simulink model "PassengerCar"  (R2019b)
settings: Solver=ode1  StartTime=0  StopTime=25  FixedStep=1.0000000000000000e-003  RelTol=1e-3
InitFcn:
  | sampleTime = str2double(get_param(bdroot, 'FixedStep'));
undefined symbols (not defined in the file or in its folder): AccPedalPos, BrakePedalPos, BrakeSwitch, DiscIntNeverNeededParam, DYNA4, EngSpd, IgnitionSwitch, InitialGear, InitialSpeed, IntendedEngTrq, LeftIndicator, MainBrakePress, MaxGear, MDL, MinGear, RefAcc, RefLane, RefLatPos, RefPath, RefPathCurv, RefSpd, RefSpdPreview, RefSpdRetrospect, RightIndicator, SteeringWheelAng, SteeringWheelTrq, UserDefinedRefValue, vm_const
libraries: UtilitiesLibrary x31, simulink x18, WheelSystemModules x13, LongitudinalControllerModules x13, LateralControllerModules x7, AnimationBusselectorModules x5, EnvironmentModules x5, BasicEngineControlModules x5, MiscellaneousControlModules x5, Animation3Modules x4, AuxiliariesModules x4, TireModules x4
(part 38 of 39)

== system PassengerCar/Vehicle/Drivetrain/DrivetrainPhysics/DrivetrainPhysicsOutputs/Rear3RightShaftOutput/Rear3RightShaftOutput ==
  Trq[Nm]___UNIQUE_1 : Inport  Description=|  PortDimensions=[1]
      | <name>Trq[Nm]</name>
      | <comment></comment>
  RotSpdDifferentialOut[rad/s]___UNIQUE_1 : Inport  Description=|  Port=2  PortDimensions=[1]
      | <name>RotSpdDifferentialOut[rad/s]</name>
      | <comment></comment>
  RotAcc[rad/s**2]___UNIQUE_1 : Inport  Description=|  Port=3  PortDimensions=[1]
      | <name>RotAcc[rad/s**2]</name>
      | <comment></comment>
  DerivativeOfTrq_wrt_RotAng[Nm/rad]___UNIQUE_1 : Inport  Description=|  Port=4  PortDimensions=[1]
      | <name>DerivativeOfTrq_wrt_RotAng[Nm/rad]</name>
      | <comment></comment>
  DerivativeOfTrq_wrt_WheelSpd[Nm/(rad/s)]___UNIQUE_1 : Inport  Description=|  Port=5  PortDimensions=[1]
      | <name>DerivativeOfTrq_wrt_WheelSpd[Nm/(rad/s)]</name>
      | <comment></comment>
  AddInrt[kg*m**2]___UNIQUE_1 : Inport  Description=|  Port=6  PortDimensions=[1]
      | <name>AddInrt[kg*m**2]</name>
      | <comment></comment>
  FrictionTrq[Nm]___UNIQUE_1 : Inport  Description=|  Port=7  PortDimensions=[1]
      | <name>FrictionTrq[Nm]</name>
      | <comment></comment>
  __TDD__Rear3RightShaft.AddInrt[kg*m**2] : Demux  Outputs=[1]
  __TDD__Rear3RightShaft.DerivativeOfTrq_wrt_RotAng[Nm/rad] : Demux  Outputs=[1]
  __TDD__Rear3RightShaft.DerivativeOfTrq_wrt_WheelSpd[Nm/(rad/s)] : Demux  Outputs=[1]
  __TDD__Rear3RightShaft.FrictionTrq[Nm] : Demux  Outputs=[1]
  __TDD__Rear3RightShaft.RotAcc[rad/s**2] : Demux  Outputs=[1]
  __TDD__Rear3RightShaft.RotSpdDifferentialOut[rad/s] : Demux  Outputs=[1]
  __TDD__Rear3RightShaft.Trq[Nm] : Demux  Outputs=[1]
  __TDO__Rear3RightShaft : BusCreator  Inputs=7
  Rear3RightShaft___UNIQUE_1 : Outport  Description=|  PortDimensions=[7]  VectorParamsAs1DForOutWhenUnconnected=off
      | <name>Trq[Nm]</name>
      | <comment></comment>
  wires:
  Trq[Nm]___UNIQUE_1/1 -> __TDD__Rear3RightShaft.Trq[Nm]/1
  __TDD__Rear3RightShaft.Trq[Nm]/1 -> __TDO__Rear3RightShaft/1  "Trq[Nm]"
  RotSpdDifferentialOut[rad/s]___UNIQUE_1/1 -> __TDD__Rear3RightShaft.RotSpdDifferentialOut[rad/s]/1
  __TDD__Rear3RightShaft.RotSpdDifferentialOut[rad/s]/1 -> __TDO__Rear3RightShaft/2  "RotSpdDifferentialOut[rad/s]"
  RotAcc[rad/s**2]___UNIQUE_1/1 -> __TDD__Rear3RightShaft.RotAcc[rad/s**2]/1
  __TDD__Rear3RightShaft.RotAcc[rad/s**2]/1 -> __TDO__Rear3RightShaft/3  "RotAcc[rad/s**2]"
  DerivativeOfTrq_wrt_RotAng[Nm/rad]___UNIQUE_1/1 -> __TDD__Rear3RightShaft.DerivativeOfTrq_wrt_RotAng[Nm/rad]/1
  __TDD__Rear3RightShaft.DerivativeOfTrq_wrt_RotAng[Nm/rad]/1 -> __TDO__Rear3RightShaft/4  "DerivativeOfTrq_wrt_RotAng[Nm/rad]"
  DerivativeOfTrq_wrt_WheelSpd[Nm/(rad/s)]___UNIQUE_1/1 -> __TDD__Rear3RightShaft.DerivativeOfTrq_wrt_WheelSpd[Nm/(rad/s)]/1
  __TDD__Rear3RightShaft.DerivativeOfTrq_wrt_WheelSpd[Nm/(rad/s)]/1 -> __TDO__Rear3RightShaft/5  "DerivativeOfTrq_wrt_WheelSpd[Nm/(rad/s)]"
  AddInrt[kg*m**2]___UNIQUE_1/1 -> __TDD__Rear3RightShaft.AddInrt[kg*m**2]/1
  __TDD__Rear3RightShaft.AddInrt[kg*m**2]/1 -> __TDO__Rear3RightShaft/6  "AddInrt[kg*m**2]"
  FrictionTrq[Nm]___UNIQUE_1/1 -> __TDD__Rear3RightShaft.FrictionTrq[Nm]/1
  __TDD__Rear3RightShaft.FrictionTrq[Nm]/1 -> __TDO__Rear3RightShaft/7  "FrictionTrq[Nm]"
  __TDO__Rear3RightShaft/1 -> Rear3RightShaft___UNIQUE_1/1  "Rear3RightShaft"

== system PassengerCar/Vehicle/Drivetrain/DrivetrainPhysics/DrivetrainPhysicsOutputs/RearDifferentialOutput/RearDifferentialOutput ==
  InSpd[rad/s]___UNIQUE_1 : Inport  Description=|  PortDimensions=[1]
      | <name>InSpd[rad/s]</name>
      | <comment></comment>
  LeftOutCutTrq[Nm]___UNIQUE_1 : Inport  Description=|  Port=2  PortDimensions=[1]
      | <name>LeftOutCutTrq[Nm]</name>
      | <comment></comment>
  RightOutCutTrq[Nm]___UNIQUE_1 : Inport  Description=|  Port=3  PortDimensions=[1]
      | <name>RightOutCutTrq[Nm]</name>
      | <comment></comment>
  LossPower[W]___UNIQUE_1 : Inport  Description=|  Port=4  PortDimensions=[1]
      | <name>LossPower[W]</name>
      | <comment></comment>
  __TDD__RearDifferential.InSpd[rad/s] : Demux  Outputs=[1]
  __TDD__RearDifferential.LeftOutCutTrq[Nm] : Demux  Outputs=[1]
  __TDD__RearDifferential.LossPower[W] : Demux  Outputs=[1]
  __TDD__RearDifferential.RightOutCutTrq[Nm] : Demux  Outputs=[1]
  __TDO__RearDifferential : BusCreator  Inputs=4
  RearDifferential___UNIQUE_1 : Outport  Description=|  PortDimensions=[4]  VectorParamsAs1DForOutWhenUnconnected=off
      | <name>InSpd[rad/s]</name>
      | <comment></comment>
  wires:
  InSpd[rad/s]___UNIQUE_1/1 -> __TDD__RearDifferential.InSpd[rad/s]/1
  __TDD__RearDifferential.InSpd[rad/s]/1 -> __TDO__RearDifferential/1  "InSpd[rad/s]"
  LeftOutCutTrq[Nm]___UNIQUE_1/1 -> __TDD__RearDifferential.LeftOutCutTrq[Nm]/1
  __TDD__RearDifferential.LeftOutCutTrq[Nm]/1 -> __TDO__RearDifferential/2  "LeftOutCutTrq[Nm]"
  RightOutCutTrq[Nm]___UNIQUE_1/1 -> __TDD__RearDifferential.RightOutCutTrq[Nm]/1
  __TDD__RearDifferential.RightOutCutTrq[Nm]/1 -> __TDO__RearDifferential/3  "RightOutCutTrq[Nm]"
  LossPower[W]___UNIQUE_1/1 -> __TDD__RearDifferential.LossPower[W]/1
  __TDD__RearDifferential.LossPower[W]/1 -> __TDO__RearDifferential/4  "LossPower[W]"
  __TDO__RearDifferential/1 -> RearDifferential___UNIQUE_1/1  "RearDifferential"

== system PassengerCar/Vehicle/Drivetrain/DrivetrainPhysics/DrivetrainPhysicsOutputs/RearLeftShaftOutput/RearLeftShaftOutput ==
  Trq[Nm]___UNIQUE_1 : Inport  Description=|  PortDimensions=[1]
      | <name>Trq[Nm]</name>
      | <comment></comment>
  RotSpdDifferentialOut[rad/s]___UNIQUE_1 : Inport  Description=|  Port=2  PortDimensions=[1]
      | <name>RotSpdDifferentialOut[rad/s]</name>
      | <comment></comment>
  RotAcc[rad/s**2]___UNIQUE_1 : Inport  Description=|  Port=3  PortDimensions=[1]
      | <name>RotAcc[rad/s**2]</name>
      | <comment></comment>
  DerivativeOfTrq_wrt_RotAng[Nm/rad]___UNIQUE_1 : Inport  Description=|  Port=4  PortDimensions=[1]
      | <name>DerivativeOfTrq_wrt_RotAng[Nm/rad]</name>
      | <comment></comment>
  DerivativeOfTrq_wrt_WheelSpd[Nm/(rad/s)]___UNIQUE_1 : Inport  Description=|  Port=5  PortDimensions=[1]
      | <name>DerivativeOfTrq_wrt_WheelSpd[Nm/(rad/s)]</name>
      | <comment></comment>
  AddInrt[kg*m**2]___UNIQUE_1 : Inport  Description=|  Port=6  PortDimensions=[1]
      | <name>AddInrt[kg*m**2]</name>
      | <comment></comment>
  FrictionTrq[Nm]___UNIQUE_1 : Inport  Description=|  Port=7  PortDimensions=[1]
      | <name>FrictionTrq[Nm]</name>
      | <comment></comment>
  __TDD__RearLeftShaft.AddInrt[kg*m**2] : Demux  Outputs=[1]
  __TDD__RearLeftShaft.DerivativeOfTrq_wrt_RotAng[Nm/rad] : Demux  Outputs=[1]
  __TDD__RearLeftShaft.DerivativeOfTrq_wrt_WheelSpd[Nm/(rad/s)] : Demux  Outputs=[1]
  __TDD__RearLeftShaft.FrictionTrq[Nm] : Demux  Outputs=[1]
  __TDD__RearLeftShaft.RotAcc[rad/s**2] : Demux  Outputs=[1]
  __TDD__RearLeftShaft.RotSpdDifferentialOut[rad/s] : Demux  Outputs=[1]
  __TDD__RearLeftShaft.Trq[Nm] : Demux  Outputs=[1]
  __TDO__RearLeftShaft : BusCreator  Inputs=7
  RearLeftShaft___UNIQUE_1 : Outport  Description=|  PortDimensions=[7]  VectorParamsAs1DForOutWhenUnconnected=off
      | <name>Trq[Nm]</name>
      | <comment></comment>
  wires:
  Trq[Nm]___UNIQUE_1/1 -> __TDD__RearLeftShaft.Trq[Nm]/1
  __TDD__RearLeftShaft.Trq[Nm]/1 -> __TDO__RearLeftShaft/1  "Trq[Nm]"
  RotSpdDifferentialOut[rad/s]___UNIQUE_1/1 -> __TDD__RearLeftShaft.RotSpdDifferentialOut[rad/s]/1
  __TDD__RearLeftShaft.RotSpdDifferentialOut[rad/s]/1 -> __TDO__RearLeftShaft/2  "RotSpdDifferentialOut[rad/s]"
  RotAcc[rad/s**2]___UNIQUE_1/1 -> __TDD__RearLeftShaft.RotAcc[rad/s**2]/1
  __TDD__RearLeftShaft.RotAcc[rad/s**2]/1 -> __TDO__RearLeftShaft/3  "RotAcc[rad/s**2]"
  DerivativeOfTrq_wrt_RotAng[Nm/rad]___UNIQUE_1/1 -> __TDD__RearLeftShaft.DerivativeOfTrq_wrt_RotAng[Nm/rad]/1
  __TDD__RearLeftShaft.DerivativeOfTrq_wrt_RotAng[Nm/rad]/1 -> __TDO__RearLeftShaft/4  "DerivativeOfTrq_wrt_RotAng[Nm/rad]"
  DerivativeOfTrq_wrt_WheelSpd[Nm/(rad/s)]___UNIQUE_1/1 -> __TDD__RearLeftShaft.DerivativeOfTrq_wrt_WheelSpd[Nm/(rad/s)]/1
  __TDD__RearLeftShaft.DerivativeOfTrq_wrt_WheelSpd[Nm/(rad/s)]/1 -> __TDO__RearLeftShaft/5  "DerivativeOfTrq_wrt_WheelSpd[Nm/(rad/s)]"
  AddInrt[kg*m**2]___UNIQUE_1/1 -> __TDD__RearLeftShaft.AddInrt[kg*m**2]/1
  __TDD__RearLeftShaft.AddInrt[kg*m**2]/1 -> __TDO__RearLeftShaft/6  "AddInrt[kg*m**2]"
  FrictionTrq[Nm]___UNIQUE_1/1 -> __TDD__RearLeftShaft.FrictionTrq[Nm]/1
  __TDD__RearLeftShaft.FrictionTrq[Nm]/1 -> __TDO__RearLeftShaft/7  "FrictionTrq[Nm]"
  __TDO__RearLeftShaft/1 -> RearLeftShaft___UNIQUE_1/1  "RearLeftShaft"

== system PassengerCar/Vehicle/Drivetrain/DrivetrainPhysics/DrivetrainPhysicsOutputs/RearRightShaftOutput/RearRightShaftOutput ==
  Trq[Nm]___UNIQUE_1 : Inport  Description=|  PortDimensions=[1]
      | <name>Trq[Nm]</name>
      | <comment></comment>
  RotSpdDifferentialOut[rad/s]___UNIQUE_1 : Inport  Description=|  Port=2  PortDimensions=[1]
      | <name>RotSpdDifferentialOut[rad/s]</name>
      | <comment></comment>
  RotAcc[rad/s**2]___UNIQUE_1 : Inport  Description=|  Port=3  PortDimensions=[1]
      | <name>RotAcc[rad/s**2]</name>
      | <comment></comment>
  DerivativeOfTrq_wrt_RotAng[Nm/rad]___UNIQUE_1 : Inport  Description=|  Port=4  PortDimensions=[1]
      | <name>DerivativeOfTrq_wrt_RotAng[Nm/rad]</name>
      | <comment></comment>
  DerivativeOfTrq_wrt_WheelSpd[Nm/(rad/s)]___UNIQUE_1 : Inport  Description=|  Port=5  PortDimensions=[1]
      | <name>DerivativeOfTrq_wrt_WheelSpd[Nm/(rad/s)]</name>
      | <comment></comment>
  AddInrt[kg*m**2]___UNIQUE_1 : Inport  Description=|  Port=6  PortDimensions=[1]
      | <name>AddInrt[kg*m**2]</name>
      | <comment></comment>
  FrictionTrq[Nm]___UNIQUE_1 : Inport  Description=|  Port=7  PortDimensions=[1]
      | <name>FrictionTrq[Nm]</name>
      | <comment></comment>
  __TDD__RearRightShaft.AddInrt[kg*m**2] : Demux  Outputs=[1]
  __TDD__RearRightShaft.DerivativeOfTrq_wrt_RotAng[Nm/rad] : Demux  Outputs=[1]
  __TDD__RearRightShaft.DerivativeOfTrq_wrt_WheelSpd[Nm/(rad/s)] : Demux  Outputs=[1]
  __TDD__RearRightShaft.FrictionTrq[Nm] : Demux  Outputs=[1]
  __TDD__RearRightShaft.RotAcc[rad/s**2] : Demux  Outputs=[1]
  __TDD__RearRightShaft.RotSpdDifferentialOut[rad/s] : Demux  Outputs=[1]
  __TDD__RearRightShaft.Trq[Nm] : Demux  Outputs=[1]
  __TDO__RearRightShaft : BusCreator  Inputs=7
  RearRightShaft___UNIQUE_1 : Outport  Description=|  PortDimensions=[7]  VectorParamsAs1DForOutWhenUnconnected=off
      | <name>Trq[Nm]</name>
      | <comment></comment>
  wires:
  Trq[Nm]___UNIQUE_1/1 -> __TDD__RearRightShaft.Trq[Nm]/1
  __TDD__RearRightShaft.Trq[Nm]/1 -> __TDO__RearRightShaft/1  "Trq[Nm]"
  RotSpdDifferentialOut[rad/s]___UNIQUE_1/1 -> __TDD__RearRightShaft.RotSpdDifferentialOut[rad/s]/1
  __TDD__RearRightShaft.RotSpdDifferentialOut[rad/s]/1 -> __TDO__RearRightShaft/2  "RotSpdDifferentialOut[rad/s]"
  RotAcc[rad/s**2]___UNIQUE_1/1 -> __TDD__RearRightShaft.RotAcc[rad/s**2]/1
  __TDD__RearRightShaft.RotAcc[rad/s**2]/1 -> __TDO__RearRightShaft/3  "RotAcc[rad/s**2]"
  DerivativeOfTrq_wrt_RotAng[Nm/rad]___UNIQUE_1/1 -> __TDD__RearRightShaft.DerivativeOfTrq_wrt_RotAng[Nm/rad]/1
  __TDD__RearRightShaft.DerivativeOfTrq_wrt_RotAng[Nm/rad]/1 -> __TDO__RearRightShaft/4  "DerivativeOfTrq_wrt_RotAng[Nm/rad]"
  DerivativeOfTrq_wrt_WheelSpd[Nm/(rad/s)]___UNIQUE_1/1 -> __TDD__RearRightShaft.DerivativeOfTrq_wrt_WheelSpd[Nm/(rad/s)]/1
  __TDD__RearRightShaft.DerivativeOfTrq_wrt_WheelSpd[Nm/(rad/s)]/1 -> __TDO__RearRightShaft/5  "DerivativeOfTrq_wrt_WheelSpd[Nm/(rad/s)]"
  AddInrt[kg*m**2]___UNIQUE_1/1 -> __TDD__RearRightShaft.AddInrt[kg*m**2]/1
  __TDD__RearRightShaft.AddInrt[kg*m**2]/1 -> __TDO__RearRightShaft/6  "AddInrt[kg*m**2]"
  FrictionTrq[Nm]___UNIQUE_1/1 -> __TDD__RearRightShaft.FrictionTrq[Nm]/1
  __TDD__RearRightShaft.FrictionTrq[Nm]/1 -> __TDO__RearRightShaft/7  "FrictionTrq[Nm]"
  __TDO__RearRightShaft/1 -> RearRightShaft___UNIQUE_1/1  "RearRightShaft"

== system PassengerCar/Vehicle/Drivetrain/DrivetrainPhysics/DrivetrainPhysicsOutputs/TransferCaseOutput/TransferCaseOutput ==
  InSpd[rad/s]___UNIQUE_1 : Inport  Description=|  PortDimensions=[1]
      | <name>InSpd[rad/s]</name>
      | <comment></comment>
  FrontOutCutTrq[Nm]___UNIQUE_1 : Inport  Description=|  Port=2  PortDimensions=[1]
      | <name>FrontOutCutTrq[Nm]</name>
      | <comment></comment>
  RearOutCutTrq[Nm]___UNIQUE_1 : Inport  Description=|  Port=3  PortDimensions=[1]
      | <name>RearOutCutTrq[Nm]</name>
      | <comment></comment>
  LossPower[W]___UNIQUE_1 : Inport  Description=|  Port=4  PortDimensions=[1]
      | <name>LossPower[W]</name>
      | <comment></comment>
  __TDD__TransferCase.FrontOutCutTrq[Nm] : Demux  Outputs=[1]
  __TDD__TransferCase.InSpd[rad/s] : Demux  Outputs=[1]
  __TDD__TransferCase.LossPower[W] : Demux  Outputs=[1]
  __TDD__TransferCase.RearOutCutTrq[Nm] : Demux  Outputs=[1]
  __TDO__TransferCase : BusCreator  Inputs=4
  TransferCase___UNIQUE_1 : Outport  Description=|  PortDimensions=[4]  VectorParamsAs1DForOutWhenUnconnected=off
      | <name>InSpd[rad/s]</name>
      | <comment></comment>
  wires:
  InSpd[rad/s]___UNIQUE_1/1 -> __TDD__TransferCase.InSpd[rad/s]/1
  __TDD__TransferCase.InSpd[rad/s]/1 -> __TDO__TransferCase/1  "InSpd[rad/s]"
  FrontOutCutTrq[Nm]___UNIQUE_1/1 -> __TDD__TransferCase.FrontOutCutTrq[Nm]/1
  __TDD__TransferCase.FrontOutCutTrq[Nm]/1 -> __TDO__TransferCase/2  "FrontOutCutTrq[Nm]"
  RearOutCutTrq[Nm]___UNIQUE_1/1 -> __TDD__TransferCase.RearOutCutTrq[Nm]/1
  __TDD__TransferCase.RearOutCutTrq[Nm]/1 -> __TDO__TransferCase/3  "RearOutCutTrq[Nm]"
  LossPower[W]___UNIQUE_1/1 -> __TDD__TransferCase.LossPower[W]/1
  __TDD__TransferCase.LossPower[W]/1 -> __TDO__TransferCase/4  "LossPower[W]"
  __TDO__TransferCase/1 -> TransferCase___UNIQUE_1/1  "TransferCase"

== system PassengerCar/Vehicle/Drivetrain/DrivetrainPhysics/DrivetrainPhysicsOutputs/TransmissionOutput/TransmissionOutput ==
  NumFwdGears[-]___UNIQUE_1 : Inport  Description=|  PortDimensions=[1]
      | <name>NumFwdGears[-]</name>
      | <comment></comment>
  Type[-]___UNIQUE_1 : Inport  Description=|  Port=2  PortDimensions=[1]
      | <name>Type[-]</name>
      | <comment></comment>
  Gear[-4;20]___UNIQUE_1 : Inport  Description=|  Port=3  PortDimensions=[1]
      | <name>Gear[-4;20]</name>
      | <comment></comment>
  InSpd[rad/s]___UNIQUE_1 : Inport  Description=|  Port=4  PortDimensions=[1]
      | <name>InSpd[rad/s]</name>
      | <comment></comment>
  OutSpd[rad/s]___UNIQUE_1 : Inport  Description=|  Port=5  PortDimensions=[1]
      | <name>OutSpd[rad/s]</name>
      | <comment></comment>
  GearChangeTimeConst[s]___UNIQUE_1 : Inport  Description=|  Port=6  PortDimensions=[1]
      | <name>GearChangeTimeConst[s]</name>
      | <comment></comment>
  OutCutTrq[Nm]___UNIQUE_1 : Inport  Description=|  Port=7  PortDimensions=[1]
      | <name>OutCutTrq[Nm]</name>
      | <comment></comment>
  LossPower[W]___UNIQUE_1 : Inport  Description=|  Port=8  PortDimensions=[1]
      | <name>LossPower[W]</name>
      | <comment></comment>
  TurbTrq[Nm]___UNIQUE_1 : Inport  Description=|  Port=9  PortDimensions=[1]
      | <name>TurbTrq[Nm]</name>
      | <comment></comment>
  LockUpClutchPos[0_1]___UNIQUE_1 : Inport  Description=|  Port=10  PortDimensions=[1]
      | <name>LockUpClutchPos[0_1]</name>
      | <comment></comment>
  __TDD__Transmission.GearChangeTimeConst[s] : Demux  Outputs=[1]
  __TDD__Transmission.Gear[-4;20] : Demux  Outputs=[1]
  __TDD__Transmission.InSpd[rad/s] : Demux  Outputs=[1]
  __TDD__Transmission.LockUpClutchPos[0_1] : Demux  Outputs=[1]
  __TDD__Transmission.LossPower[W] : Demux  Outputs=[1]
  __TDD__Transmission.NumFwdGears[-] : Demux  Outputs=[1]
  __TDD__Transmission.OutCutTrq[Nm] : Demux  Outputs=[1]
  __TDD__Transmission.OutSpd[rad/s] : Demux  Outputs=[1]
  __TDD__Transmission.TurbTrq[Nm] : Demux  Outputs=[1]
  __TDD__Transmission.Type[-] : Demux  Outputs=[1]
  __TDO__Transmission : BusCreator  Inputs=10
  Transmission___UNIQUE_1 : Outport  Description=|  PortDimensions=[10]  VectorParamsAs1DForOutWhenUnconnected=off
      | <name>NumFwdGears[-]</name>
      | <comment></comment>
  wires:
  NumFwdGears[-]___UNIQUE_1/1 -> __TDD__Transmission.NumFwdGears[-]/1
  __TDD__Transmission.NumFwdGears[-]/1 -> __TDO__Transmission/1  "NumFwdGears[-]"
  Type[-]___UNIQUE_1/1 -> __TDD__Transmission.Type[-]/1
  __TDD__Transmission.Type[-]/1 -> __TDO__Transmission/2  "Type[-]"
  Gear[-4;20]___UNIQUE_1/1 -> __TDD__Transmission.Gear[-4;20]/1
  __TDD__Transmission.Gear[-4;20]/1 -> __TDO__Transmission/3  "Gear[-4;20]"
  InSpd[rad/s]___UNIQUE_1/1 -> __TDD__Transmission.InSpd[rad/s]/1
  __TDD__Transmission.InSpd[rad/s]/1 -> __TDO__Transmission/4  "InSpd[rad/s]"
  OutSpd[rad/s]___UNIQUE_1/1 -> __TDD__Transmission.OutSpd[rad/s]/1
  __TDD__Transmission.OutSpd[rad/s]/1 -> __TDO__Transmission/5  "OutSpd[rad/s]"
  GearChangeTimeConst[s]___UNIQUE_1/1 -> __TDD__Transmission.GearChangeTimeConst[s]/1
  __TDD__Transmission.GearChangeTimeConst[s]/1 -> __TDO__Transmission/6  "GearChangeTimeConst[s]"
  OutCutTrq[Nm]___UNIQUE_1/1 -> __TDD__Transmission.OutCutTrq[Nm]/1
  __TDD__Transmission.OutCutTrq[Nm]/1 -> __TDO__Transmission/7  "OutCutTrq[Nm]"
  LossPower[W]___UNIQUE_1/1 -> __TDD__Transmission.LossPower[W]/1
  __TDD__Transmission.LossPower[W]/1 -> __TDO__Transmission/8  "LossPower[W]"
  TurbTrq[Nm]___UNIQUE_1/1 -> __TDD__Transmission.TurbTrq[Nm]/1
  __TDD__Transmission.TurbTrq[Nm]/1 -> __TDO__Transmission/9  "TurbTrq[Nm]"
  LockUpClutchPos[0_1]___UNIQUE_1/1 -> __TDD__Transmission.LockUpClutchPos[0_1]/1
  __TDD__Transmission.LockUpClutchPos[0_1]/1 -> __TDO__Transmission/10  "LockUpClutchPos[0_1]"
  __TDO__Transmission/1 -> Transmission___UNIQUE_1/1  "Transmission"

== system PassengerCar/VehicleControl/LateralControl/Disabled LateralControl/ControlSystems/Control Systems Parameters/CurvatureControl ==
  DynaModuleInfo : Subsystem  Tag=DynaModuleInfo
      mask init:
      | data = get_param(gcb, 'UserData');
      mask Display: disp(['Type = ', data.type, '\nName = ', char(data.name)]);

== system PassengerCar/VehicleControl/LateralControl/Disabled LateralControl/ControlSystems/Control Systems Parameters/PathControl ==
  DynaModuleInfo : Subsystem  Tag=DynaModuleInfo
      mask init:
      | data = get_param(gcb, 'UserData');
      mask Display: disp(['Type = ', data.type, '\nName = ', char(data.name)]);

== system PassengerCar/VehicleControl/LateralControl/Disabled LateralControl/ControlSystems/Lateral Controller/User-Defined Control ==
  UserDefinedControl : Subsystem
      settings: CopyFcn=DYNA4.Internal.ModelCallbacks.Modules.UpdateMaskParameters(gcb);  DeleteFcn=dm_close_block_mask  ModelCloseFcn=dm_close_block_mask  NameChangeFcn=DYNA4.Internal.ModelCallbacks.Modules.UpdateMaskParameters(gcb);  OpenFcn=dm_open_block_mask('vm_dflt_vehiclecontrol_user_defined_lateral_control');

== system PassengerCar/VehicleControl/LateralControl/Disabled LateralControl/ControlSystemsPreprocessor/Maneuver/DynaModuleInfo ==

== system PassengerCar/VehicleControl/LateralControl/Enabled LateralControl/ControlSystems/Lateral Controller/Initialization ==
  Action Port : ActionPort  InitializeStates=reset  PropagateVarSize=During execution  ActionPortLabel=default:
  Bus Creator : BusCreator  Inputs=3
  Constant : Constant  Value=0
  Constant1 : Constant  Value=0
  Constant2 : Constant  Value=0
  SteeringWheelDemands : Outport  VectorParamsAs1DForOutWhenUnconnected=off
  wires:
  Constant2/1 -> Bus Creator/3  "SteeringWheelInputSwitch[-]"
  Constant1/1 -> Bus Creator/2  "SteeringWheelTrq[Nm]"
  Bus Creator/1 -> SteeringWheelDemands/1
  Constant/1 -> Bus Creator/1  "SteeringWheelAng[rad]"

== system PassengerCar/VehicleControl/LateralControl/Enabled LateralControl/ControlSystems/Lateral Controller/Path and Curvature Control ==
  ControlInputs : Inport
  ControllerParameters : Inport  Port=2
  VehicleInfo : Inport  Port=3
  Action Port : ActionPort  InitializeStates=reset  PropagateVarSize=During execution  ActionPortLabel=case [ 3 4 ]:
  Bus Creator : BusCreator  Inputs=3
  Bus Selector1 : BusSelector  OutputSignals=Chassis_FrontAxle_Steering_SteeringWheelTrq[Nm]
  Constant1 : Constant  Value=0
  Gain : Gain
  PathControl : LateralControllerModules/PathControl  Tag=vedynaPathCtrlMask  local_comp_inst=1  system_comp_inst=1  sample_time=-1
  required by merge block : SignalConversion  OverrideOpt=off
  SteeringWheelDemands : Outport  VectorParamsAs1DForOutWhenUnconnected=off
  wires:
  Gain/1 -> Bus Creator/2  "SteeringWheelTrq[Nm]"
  Bus Selector1/1 -> Gain/1  "<Chassis_FrontAxle_Steering_SteeringWheelTrq[Nm]>"
  required by merge block/1 -> Bus Creator/1  "SteeringWheelAng[rad]"
  Constant1/1 -> Bus Creator/3  "SteeringWheelInputSwitch[-]"
  Bus Creator/1 -> SteeringWheelDemands/1
  PathControl/1 -> required by merge block/1
  ControllerParameters/1 -> PathControl/2
  ControlInputs/1 -> PathControl/1
  VehicleInfo/1 -> PathControl/3, Bus Selector1/1

== system PassengerCar/VehicleControl/LateralControl/Enabled LateralControl/ControlSystems/Lateral Controller/Steering Wheel Angle Input ==
  ControlInputs : Inport
  VehicleInfo : Inport  Port=2
  Action Port : ActionPort  InitializeStates=reset  PropagateVarSize=During execution  ActionPortLabel=case [ 1 ]:
  Bus Creator : BusCreator  Inputs=3
  Bus Selector : BusSelector  OutputSignals=SteeringWheelAng
  Bus Selector1 : BusSelector  OutputSignals=Chassis_FrontAxle_Steering_SteeringWheelTrq[Nm]
  Constant1 : Constant  Value=0
  Gain : Gain
  required by merge block : SignalConversion  OverrideOpt=off
  SteeringWheelDemands : Outport  VectorParamsAs1DForOutWhenUnconnected=off
  wires:
  Gain/1 -> Bus Creator/2  "SteeringWheelTrq[Nm]"
  VehicleInfo/1 -> Bus Selector1/1
  Constant1/1 -> Bus Creator/3  "SteeringWheelInputSwitch[-]"
  Bus Selector1/1 -> Gain/1  "<Chassis_FrontAxle_Steering_SteeringWheelTrq[Nm]>"
  Bus Creator/1 -> SteeringWheelDemands/1
  required by merge block/1 -> Bus Creator/1  "SteeringWheelAng[rad]"
  Bus Selector/1 -> required by merge block/1  "<SteeringWheelAng>"
  ControlInputs/1 -> Bus Selector/1

== system PassengerCar/VehicleControl/LateralControl/Enabled LateralControl/ControlSystems/Lateral Controller/Steering Wheel Torque Input ==
  ControlInputs : Inport
  VehicleInfo : Inport  Port=2
  Action Port : ActionPort  InitializeStates=reset  PropagateVarSize=During execution  ActionPortLabel=case [ 2 ]:
  Bus Creator : BusCreator  Inputs=3
  Bus Selector : BusSelector  OutputSignals=SteeringWheelTrq
  Bus Selector1 : BusSelector  OutputSignals=Chassis_FrontAxle_Steering_SteeringWheelAng[rad]
  Constant1 : Constant
  Gain : Gain
  required by merge block : SignalConversion  OverrideOpt=off
  SteeringWheelDemands : Outport  VectorParamsAs1DForOutWhenUnconnected=off
  wires:
  Gain/1 -> Bus Creator/1  "SteeringWheelAng[rad]"
  required by merge block/1 -> Bus Creator/2  "SteeringWheelTrq[Nm]"
  VehicleInfo/1 -> Bus Selector1/1
  Bus Selector/1 -> required by merge block/1  "<SteeringWheelTrq>"
  ControlInputs/1 -> Bus Selector/1
  Bus Selector1/1 -> Gain/1  "<Chassis_FrontAxle_Steering_SteeringWheelAng[rad]>"
  Bus Creator/1 -> SteeringWheelDemands/1
  Constant1/1 -> Bus Creator/3  "SteeringWheelInputSwitch[-]"

== system PassengerCar/VehicleControl/LateralControl/Enabled LateralControl/ControlSystems/Lateral Controller/User-Defined Control ==
  ControlInputs : Inport
  VehicleInfo : Inport  Port=2
  SourceIdentifiers : Inport  Port=3
  SubtaskIdentifiers : Inport  Port=4
  Action Port : ActionPort  InitializeStates=reset  PropagateVarSize=During execution  ActionPortLabel=case [ 5 ]:
  Bus Creator : BusCreator  Inputs=3
  Bus Selector1 : BusSelector  OutputSignals=UserDefinedRefValue
  Bus Selector2 : BusSelector  OutputSignals=Chassis_FrontAxle_Steering_SteeringWheelTrq[Nm]
  Constant1 : Constant  Value=0
  Gain : Gain
  UserDefinedControl : LateralControllerModules/UserDefinedLateralControl  DATA_NODE=MDL.VehicleControl.LateralControl.ControlSystems.UserDefinedControl  SteeringWheelAngle=MDL.VehicleControl.LateralControl.ControlSystems.UserDefinedControl.SteeringWheelAng
  SteeringWheelDemands : Outport  VectorParamsAs1DForOutWhenUnconnected=off
  UserDefinedRefValue[-] : Outport  Port=2  PortDimensions=1  OutputWhenDisabled=reset  InitialOutput=0  VectorParamsAs1DForOutWhenUnconnected=off
  wires:
  Gain/1 -> Bus Creator/2  "SteeringWheelTrq[Nm]"
  Bus Selector2/1 -> Gain/1  "<Chassis_FrontAxle_Steering_SteeringWheelTrq[Nm]>"
  Constant1/1 -> Bus Creator/3  "SteeringWheelInputSwitch[-]"
  Bus Creator/1 -> SteeringWheelDemands/1
  UserDefinedControl/1 -> Bus Creator/1  "SteeringWheelAng[rad]"
  Bus Selector1/1 -> UserDefinedRefValue[-]/1  "<UserDefinedRefValue>"
  SubtaskIdentifiers/1 -> UserDefinedControl/1
  VehicleInfo/1 -> UserDefinedControl/4, Bus Selector2/1
  SourceIdentifiers/1 -> UserDefinedControl/2
  ControlInputs/1 -> Bus Selector1/1, UserDefinedControl/3

== system PassengerCar/VehicleControl/LateralControl/Enabled LateralControl/ControlSystemsPreprocessor/External Presetting of Controller /Presetting Source Identifiers ==
  note: SOURCE_NOMINALPATH = 1;
      | 	SOURCE_LANE = 2;
      | 	SOURCE_CONSTANT = 3;
      | 	SOURCE_TABLE_DISCRETE = 4;
      | 	SOURCE_TABLE_LINEAR = 5;
      | 	SOURCE_TABLE_CUBIC = 6;
      | 	SOURCE_TABLE_HAVERSINE = 7;
      | 	SOURCE_AUTOMATIC = 8;
      | 	SOURCE_SINE_TIME = 9;
      | 	SOURCE_SINE_PATH = 10;
      | 	SOURCE_HOLD = 11;
      | 	SOURCE_EXTERNAL = 12;
      | 	SOURCE_EXTERNAL_NOMINALPATH = 13;
      | 	SOURCE_EXTERNAL_LANE = 14;
  "ExternalControlVariablesEnforced " : Inport
  SourceIdentifiers : Inport  Port=2
  Bus Selector : BusSelector  OutputSignals=CTRL_LateralControl_RefPathEnforced,CTRL_LateralControl_RefLaneEnforced,CTRL_LateralControl_RefLatPosEnforced,CTRL_LateralControl_RefCurvEnforced,CTRL_LateralControl_UserDefinedRefValueEnforced
  Bus Selector6 : BusSelector  OutputSignals=RefPath,RefLane,RefLatPos,RefPathCurv,UserDefinedRefValue
  PathCtrl_Path : BusAssignment  AssignedSignals=RefPath,RefLane,RefLatPos,RefPathCurv,UserDefinedRefValue
  RefLaneExternal : Constant  Value=vm_const('SOURCE_EXTERNAL_LANE')
  RefLatPosExternal : Constant  Value=vm_const('SOURCE_EXTERNAL')
  RefPathCurvExternal : Constant  Value=vm_const('SOURCE_EXTERNAL')
  RefPathExternal : Constant  Value=vm_const('SOURCE_EXTERNAL_NOMINALPATH')
  Switch{1..2,5..7} (5 alike) : Switch  Criteria=u2 > Threshold
  UserDefinedRefValueExternal : Constant  Value=vm_const('SOURCE_EXTERNAL')
  ModifiedSourceIdentifiers : Outport  VectorParamsAs1DForOutWhenUnconnected=off
  wires:
  Bus Selector6/5 -> Switch2/3  "<UserDefinedRefValue>"
  Bus Selector6/4 -> Switch1/3  "<RefPathCurv>"
  Bus Selector6/3 -> Switch7/3  "<RefLatPos>"
  Bus Selector6/2 -> Switch6/3  "<RefLane>"
  Bus Selector6/1 -> Switch5/3  "<RefPath>"
  Switch2/1 -> PathCtrl_Path/6
  Switch1/1 -> PathCtrl_Path/5
  Switch7/1 -> PathCtrl_Path/4
  Switch6/1 -> PathCtrl_Path/3
  Switch5/1 -> PathCtrl_Path/2
  PathCtrl_Path/1 -> ModifiedSourceIdentifiers/1
  Bus Selector/5 -> Switch2/2  "<CTRL_LateralControl_UserDefinedRefValueEnforced>"
  UserDefinedRefValueExternal/1 -> Switch2/1
  RefPathCurvExternal/1 -> Switch1/1
  Bus Selector/4 -> Switch1/2  "<CTRL_LateralControl_RefCurvEnforced>"
  RefLatPosExternal/1 -> Switch7/1
  Bus Selector/3 -> Switch7/2  "<CTRL_LateralControl_RefLatPosEnforced>"
  Bus Selector/2 -> Switch6/2  "<CTRL_LateralControl_RefLaneEnforced>"
  RefLaneExternal/1 -> Switch6/1
  RefPathExternal/1 -> Switch5/1
  Bus Selector/1 -> Switch5/2  "<CTRL_LateralControl_RefPathEnforced>"
  "ExternalControlVariablesEnforced "/1 -> Bus Selector/1
  SourceIdentifiers/1 -> PathCtrl_Path/1, Bus Selector6/1

== system PassengerCar/VehicleControl/LateralControl/Enabled LateralControl/ControlSystemsPreprocessor/External Presetting of Controller /Presetting Task Identifiers ==
  TaskIdentifiers : Inport
  "ExternalControlVariablesEnforced " : Inport  Port=2
  Bus Creator : BusCreator  Inputs=2
  Bus Selector : BusSelector  OutputSignals=CTRL_LateralControl_RefPathEnforced,CTRL_LateralControl_RefLaneEnforced,CTRL_LateralControl_RefLatPosEnforced,CTRL_LateralControl_RefCurvEnforced,CTRL_LateralControl_UserDefinedRefValueEnforced  OutputAsBus=on
  Bus Selector1 : BusSelector  OutputSignals=Task[-],Subtask[-]
  Bus to Vector : BusToVector
  ChooseMax : MinMax  Function=max
  Demux : Demux  Outputs=2
  Gain : Gain  Gain=[5 4 3 2 1]
  Multiport Switch : MultiPortSwitch  DataPortOrder=Zero-based contiguous  Inputs=6  zeroidx=on
  Mux : Mux  Inputs=2
  Speed Control : Constant  Value=[vm_const('TASK_LAT_PATH_CONTROL') vm_const('SUBTASK_LAT_PATH_CONTROL_PATH')]
  Speed Control1 : Constant  Value=[vm_const('TASK_LAT_CURVATURE_CONTROL') 0]
  Speed Control2 : Constant  Value=[vm_const('TASK_LAT_USER_DEFINED') 0]
  Speed Control3 : Constant  Value=[vm_const('TASK_LAT_PATH_CONTROL') vm_const('SUBTASK_LAT_PATH_CONTROL_LANE')]
  Speed Control4 : Constant  Value=[vm_const('TASK_LAT_PATH_CONTROL') vm_const('SUBTASK_LAT_PATH_CONTROL_LATERAL_POS')]
  ModifiedTaskIdentifiers : Outport  VectorParamsAs1DForOutWhenUnconnected=off
  wires:
  Multiport Switch/1 -> Demux/1
  Speed Control2/1 -> Multiport Switch/3
  Speed Control1/1 -> Multiport Switch/4
  Speed Control4/1 -> Multiport Switch/5
  Speed Control3/1 -> Multiport Switch/6
  Speed Control/1 -> Multiport Switch/7
  Mux/1 -> Multiport Switch/2
  Gain/1 -> ChooseMax/1
  Bus to Vector/1 -> Gain/1
  Bus Selector/1 -> Bus to Vector/1
  Bus Selector1/1 -> Mux/1  "<Task[-]>"
  Bus Selector1/2 -> Mux/2  "<Subtask[-]>"
  "ExternalControlVariablesEnforced "/1 -> Bus Selector/1
  TaskIdentifiers/1 -> Bus Selector1/1
  Bus Creator/1 -> ModifiedTaskIdentifiers/1
  Demux/1 -> Bus Creator/1  "Task"
  Demux/2 -> Bus Creator/2  "Subtask"
  ChooseMax/1 -> Multiport Switch/1  "switch value"

== system PassengerCar/VehicleControl/LateralControl/Enabled LateralControl/ControlSystemsPreprocessor/Generation of Guidance Data/Initialization, SteeringWheel, UserDefined ==
  Action Port : ActionPort  InitializeStates=reset  ActionPortLabel=default:
  Constant : Constant  Value=zeros(1,7)
  TargetAndTargetAim : Outport  VectorParamsAs1DForOutWhenUnconnected=off
  wires:
  Constant/1 -> TargetAndTargetAim/1

== system PassengerCar/VehicleControl/LateralControl/Enabled LateralControl/ControlSystemsPreprocessor/Generation of Hold Data/Enabled Subsystem ==
  LatCTRL : Inport
  VehicleInfo : Inport  Port=2
  Enable : EnablePort  StatesWhenEnabling=reset  PropagateVarSize=During execution
  Bus Assignment : BusAssignment  AssignedSignals=SteeringWheelAng,SteeringWheelTrq,LeftIndicator,RightIndicator,RefLatPos,RefLane,RefPathCurv
  Bus Selector18 : BusSelector  OutputSignals=VehicleRoadInfo_RoadQ[m],VehicleRoadInfo_LaneID[-],VehicleRoadInfo_LaneCurvature[1/m]
  Bus Selector8 : BusSelector  OutputSignals=SteeringWheelAng[rad],SteeringWheelTrq[Nm],LeftIndicator[0;1],RightIndicator[0;1]
  TD_BO_LateralControlInputs all zeros : Constant  Value=0  OutDataTypeStr=Bus: TD_BO_LateralControlInputs
  HoldData : Outport  VectorParamsAs1DForOutWhenUnconnected=off
  wires:
  Bus Selector18/2 -> Bus Assignment/7  "<VehicleRoadInfo_LaneID[-]>"
  Bus Selector18/3 -> Bus Assignment/8  "<VehicleRoadInfo_LaneCurvature[1/m]>"
  Bus Selector18/1 -> Bus Assignment/6  "<VehicleRoadInfo_RoadQ[m]>"
  Bus Selector8/4 -> Bus Assignment/5  "<RightIndicator[0;1]>"
  Bus Selector8/3 -> Bus Assignment/4  "<LeftIndicator[0;1]>"
  Bus Selector8/2 -> Bus Assignment/3  "<SteeringWheelTrq[Nm]>"
  Bus Assignment/1 -> HoldData/1
  TD_BO_LateralControlInputs all zeros/1 -> Bus Assignment/1
  VehicleInfo/1 -> Bus Selector18/1
  LatCTRL/1 -> Bus Selector8/1
  Bus Selector8/1 -> Bus Assignment/2  "<SteeringWheelAng[rad]>"

== system PassengerCar/VehicleControl/LongitudinalControl/ControlSystems/Longitudinal Controller/Acceleration Control/ComputeBrakePedalPos ==
  VehicleInfo : Inport
  RefTireTrq[Nm] : Inport  Port=2
  Bus Selector : BusSelector  OutputSignals=VehicleDriverInfo_AccPedalPos[0_1]
  Calculate Brake Pedal : Subsystem
  Constant1 : Constant  Value=0
  Factor_TyreTorque_2_BrakePedalPosition : Subsystem
  no Brake AND Gas : Subsystem
  BrakePedalPos[0_1] : Outport  VectorParamsAs1DForOutWhenUnconnected=off
  wires:
  Bus Selector/1 -> no Brake AND Gas/1(AccPedal)  "<VehicleDriverInfo_AccPedalPos[0_1]>"
  VehicleInfo/1 -> Factor_TyreTorque_2_BrakePedalPosition/1(VehicleInfo), Bus Selector/1
  RefTireTrq[Nm]/1 -> Calculate Brake Pedal/2(Int Torque on Wheel)
  no Brake AND Gas/1(ModifiedBrakePedalPos [0-1]) -> BrakePedalPos[0_1]/1
  Constant1/1 -> no Brake AND Gas/3(PedalChangeTime)  "<MinPedalChangeTime[s]>"
  Calculate Brake Pedal/1(Brake Pedal Position) -> no Brake AND Gas/2(BrakePedal)
  Factor_TyreTorque_2_BrakePedalPosition/1(Factor_TyreTorque_2_BrakePedalPosition) -> Calculate Brake Pedal/1(Factor_TyreTorque_2_BrakePedalPosition)

== system PassengerCar/VehicleControl/LongitudinalControl/ControlSystems/Longitudinal Controller/Acceleration Control/ComputeIntEngTrq ==
  FeedforwardTrq[Nm] : Inport
  VehicleInfo : Inport  Port=2
  ControlTrq[Nm] : Inport  Port=3
  Avoid_Zero : Saturate  UpperLimit=inf  LowerLimit=0.1
  Bus Selector : BusSelector  OutputSignals=VehicleDriverInfo_TorqueRatio[-]
  Divide : Product  Inputs=*/
  IntTrqWheel : Sum
  Memory1 : Memory  InheritSampleTime=on
  RefTireTrq[Nm] : Outport  VectorParamsAs1DForOutWhenUnconnected=off
  RefEngTrq[Nm] : Outport  Port=2  VectorParamsAs1DForOutWhenUnconnected=off
  wires:
  Memory1/1 -> Divide/1, RefTireTrq[Nm]/1
  Avoid_Zero/1 -> Divide/2
  IntTrqWheel/1 -> Memory1/1
  Divide/1 -> RefEngTrq[Nm]/1
  Bus Selector/1 -> Avoid_Zero/1  "<VehicleDriverInfo_TorqueRatio[-]>"
  ControlTrq[Nm]/1 -> IntTrqWheel/2
  FeedforwardTrq[Nm]/1 -> IntTrqWheel/1
  VehicleInfo/1 -> Bus Selector/1

== system PassengerCar/VehicleControl/LongitudinalControl/ControlSystems/Longitudinal Controller/Acceleration Control/Write To ControlOutputs ==
  BrakePedalPos[0_1] : Inport
  IntendedEngTrq[Nm] : Inport  Port=2
  EngSpd[rad/s] : Inport  Port=3
  RefAcc[rad/s] : Inport  Port=4
  Bus Assignment : BusAssignment  AssignedSignals=BrakePedalPos,IntendedEngTrq,EngSpd,RefAcc
  Create SpeedControlOutput Bus : Constant  Value=0  OutDataTypeStr=Bus: TD_BO_LongitudinalSpeedControlOutputs
  ControlOutputs : Outport  VectorParamsAs1DForOutWhenUnconnected=off
  wires:
  Bus Assignment/1 -> ControlOutputs/1
  Create SpeedControlOutput Bus/1 -> Bus Assignment/1
  BrakePedalPos[0_1]/1 -> Bus Assignment/2
  RefAcc[rad/s]/1 -> Bus Assignment/5  "RefAcc[m/s**2]"
  EngSpd[rad/s]/1 -> Bus Assignment/4  "EngSpd[rad/s]"
  IntendedEngTrq[Nm]/1 -> Bus Assignment/3  "IntendedEngTrq[Nm]"

== system PassengerCar/VehicleControl/LongitudinalControl/ControlSystems/Longitudinal Controller/Compute Acc Pedal Position/Invert Acc Pedal ==
  VehicleInfo : Inport
  ControlOutputs : Inport  Port=2
  Action Port : ActionPort  InitializeStates=reset  PropagateVarSize=During execution  ActionPortLabel=case [ 0 2 3 4 ]:
  InvAccPedal : LongitudinalControllerModules/InvAccPedal  Tag=vedynaInvAccPedalMask  SystemSampleTime=-1  Latency=0  AutoFrameSizeCalculation=off
  ModifiedControlOutputs : Outport  VectorParamsAs1DForOutWhenUnconnected=off
  wires:
  InvAccPedal/1 -> ModifiedControlOutputs/1
  VehicleInfo/1 -> InvAccPedal/1
  ControlOutputs/1 -> InvAccPedal/2

== system PassengerCar/VehicleControl/LongitudinalControl/ControlSystems/Longitudinal Controller/Compute Acc Pedal Position/Pass Through ControlOutputs ==
  ControlOutputs : Inport
  Action Port : ActionPort  InitializeStates=reset  PropagateVarSize=During execution  ActionPortLabel=case [ 1 ]:
  ModifiedControlOutputs : Outport  VectorParamsAs1DForOutWhenUnconnected=off
  wires:
  ControlOutputs/1 -> ModifiedControlOutputs/1

== system PassengerCar/VehicleControl/LongitudinalControl/ControlSystems/Longitudinal Controller/Speed Control/Load Torque Vehicle ==
  VehSpd[m/s] : Inport
  TireRadius[m] : Inport  Port=2
  AerodynamicFrc[N] : Inport  Description=Vehicle Velocity  Port=3
  RoadSlopeLong [-] : Inport  Port=4
  SumMaxRollResistanceTrq[Nm] : Inport  Description=Vehicle Velocity  Port=5
  VehMass [kg] : Inport  Port=6
  BrakeFrc[N] : Inport  Port=7
  Constant : Constant  Value=9.81
  F_load [N] : Sum  Inputs=3  SaturateOnIntegerOverflow=on  InputSameDT=on  OutDataTypeStr=Inherit: Same as first input
  LoadTrq : Product  SaturateOnIntegerOverflow=on  InputSameDT=on  OutDataTypeStr=Inherit: Same as first input
  Resist.Torque : Product  SaturateOnIntegerOverflow=on  InputSameDT=on  OutDataTypeStr=Inherit: Same as first input
  Slope Force : Product  Inputs=3  SaturateOnIntegerOverflow=on  InputSameDT=on  OutDataTypeStr=Inherit: Same as first input
  Trigonometric Function : Trigonometry
  Trigonometric Function1 : Trigonometry  Operator=atan
  abs(F_load) [N]1 : Sum  Inputs=2  SaturateOnIntegerOverflow=on  InputSameDT=on  OutDataTypeStr=Inherit: Same as first input
  fade out load torque if speed is zero : Saturate  UpperLimit=1  LowerLimit=0
  toCompile : Subsystem  Tag=em_compile_service
      settings: AttributesFormatString=Place this block in the subsystem\n you want to compile
  LoadTrq[Nm] : Outport  VectorParamsAs1DForOutWhenUnconnected=off
  wires:
  VehSpd[m/s]/1 -> fade out load torque if speed is zero/1
  SumMaxRollResistanceTrq[Nm]/1 -> abs(F_load) [N]1/2
  TireRadius[m]/1 -> Resist.Torque/2
  Slope Force/1 -> F_load [N]/3
  Trigonometric Function/1 -> Slope Force/3
  VehMass [kg]/1 -> Slope Force/2
  Constant/1 -> Slope Force/1
  AerodynamicFrc[N]/1 -> F_load [N]/1
  BrakeFrc[N]/1 -> F_load [N]/2
  Resist.Torque/1 -> abs(F_load) [N]1/1
  RoadSlopeLong [-]/1 -> Trigonometric Function1/1
  F_load [N]/1 -> Resist.Torque/1
  abs(F_load) [N]1/1 -> LoadTrq/2
  fade out load torque if speed is zero/1 -> LoadTrq/1
  LoadTrq/1 -> LoadTrq[Nm]/1
  Trigonometric Function1/1 -> Trigonometric Function/1

== system PassengerCar/VehicleControl/LongitudinalControl/ControlSystems/Longitudinal Controller/Speed Control/Preprocessing VehicleInfo ==
  VehicleInfo : Inport
  Abs : Abs
  Add3 : Sum  Inputs=++++
  Add4 : Sum
  AverageRadius : Gain  Gain=0.25
  Bus Selector : BusSelector  OutputSignals=VehicleDriverInfo_TorqueRatio[-],VehicleDriverInfo_AccPedalPos[0_1],VehicleDriverInfo_OverallMass[kg],Chassis_VehicleBody_AbsVel[m/s],Drivetrain_DrivetrainPhysics_EngSpd[rad/s],Drivetrain_DrivetrainPhysics_Clutch_Pos[0_1],Drivetrain_DrivetrainPhysics_Transmission_Gear[-4;20],VehicleDriverInfo_TransmissionType[-],Auxiliaries_StarterTrq[Nm],VehicleDriverInfo_SumWheelRotAxisInrt[kg*m**2],Chassis_VehicleBody_AeroFrc(VehSys)[N],VehicleDriverInfo_SumMaxRollingResistanceTrq[Nm],VehicleDriverInfo_MaxDeceleration[m/s**2],WheelSystem_FrontLeft_Tire_DynamicRadius[m],WheelSystem_FrontRight_Tire_DynamicRadius[m],WheelSystem_RearLeft_Tire_DynamicRadius[m],WheelSystem_RearRight_Tire_DynamicRadius[m],VehicleDriverInfo_LongAeroDragCoeff[-],VehicleRoadInfo_RoadSlopeLong[-],VehicleDriverInfo_EngInrt[kg*m**2],VehicleDriverInfo_FullAccPedalTrq[Nm],VehicleDriverInfo_ZeroAccPedalTrq[Nm]
  DetectGearChange : Subsystem
  Product : Product  Inputs=***  RndMeth=Zero
  Product2 : Product  Inputs=**  RndMeth=Zero
  Saturation : Saturate  UpperLimit=1e6  LowerLimit=0.1
  Select x_value : Selector  InputPortWidth=3  IndexOptions=Index vector (dialog)  Indices=1  OutputSizes=1
  TractionCtrl : Subsystem
  factor from vehicle data : Gain  Gain=-1
  VehSpd[m/s] : Outport  VectorParamsAs1DForOutWhenUnconnected=off
  EngSpd[rad/s] : Outport  Port=2  VectorParamsAs1DForOutWhenUnconnected=off
  ExternalTrqs[Nm] : Outport  Port=3  VectorParamsAs1DForOutWhenUnconnected=off
  DynamicTireRadius[m] : Outport  Port=4  VectorParamsAs1DForOutWhenUnconnected=off
  VehAndWheelInrtl[kg*m**2] : Outport  Port=5  VectorParamsAs1DForOutWhenUnconnected=off
  TractionCtrlFlag[0/1] : Outport  Port=6  VectorParamsAs1DForOutWhenUnconnected=off
  MaxBrakeFrc[N] : Outport  Port=7  VectorParamsAs1DForOutWhenUnconnected=off
  FinalDriveRatio[-] : Outport  Port=8  VectorParamsAs1DForOutWhenUnconnected=off
  LongAeroDragCoeff[-] : Outport  Port=9  VectorParamsAs1DForOutWhenUnconnected=off
  AccPedalPos[0_1] : Outport  Port=10  VectorParamsAs1DForOutWhenUnconnected=off
  ClutchPos[0_1] : Outport  Port=11  VectorParamsAs1DForOutWhenUnconnected=off
  EngInrtl[kg*m**2] : Outport  Port=12  VectorParamsAs1DForOutWhenUnconnected=off
  Gear[-4;20] : Outport  Port=13  OutDataTypeStr=double  VectorParamsAs1DForOutWhenUnconnected=off
  FullAccPedalTrq[Nm] : Outport  Port=14  VectorParamsAs1DForOutWhenUnconnected=off
  ZeroAccPedalTrq[Nm] : Outport  Port=15  VectorParamsAs1DForOutWhenUnconnected=off
  AerodynamicFrc[N] : Outport  Port=16  VectorParamsAs1DForOutWhenUnconnected=off
  RoadSlopeLong[-] : Outport  Port=17  VectorParamsAs1DForOutWhenUnconnected=off
  SumMaxRollResistanceTrq[Nm] : Outport  Port=18  VectorParamsAs1DForOutWhenUnconnected=off
  VehMass[kg] : Outport  Port=19  VectorParamsAs1DForOutWhenUnconnected=off
  wires:
  Bus Selector/22 -> ZeroAccPedalTrq[Nm]/1  "<VehicleDriverInfo_ZeroAccPedalTrq[Nm]>"
  Bus Selector/21 -> FullAccPedalTrq[Nm]/1  "<VehicleDriverInfo_FullAccPedalTrq[Nm]>"
  Bus Selector/20 -> EngInrtl[kg*m**2]/1  "<VehicleDriverInfo_EngInrt[kg*m**2]>"
  VehicleInfo/1 -> Bus Selector/1
  Bus Selector/2 -> AccPedalPos[0_1]/1  "<VehicleDriverInfo_AccPedalPos[0_1]>"
  Bus Selector/7 -> Gear[-4;20]/1, DetectGearChange/1(Gear)  "<Drivetrain_DrivetrainPhysics_Transmission_Gear[-4;20]>"
  Bus Selector/8 -> DetectGearChange/2(TransmissionType)  "<VehicleDriverInfo_TransmissionType[-]>"
  Bus Selector/4 -> VehSpd[m/s]/1  "<Chassis_VehicleBody_AbsVel[m/s]>"
  Saturation/1 -> Product/3, Product/2, DynamicTireRadius[m]/1
  AverageRadius/1 -> Saturation/1
  TractionCtrl/1(ASRFlag [0/1]) -> TractionCtrlFlag[0/1]/1
  DetectGearChange/1(GearChangeFlag) -> TractionCtrl/2(GearChangeFlag [0|1])
  Product/1 -> Add4/1
  factor from vehicle data/1 -> AerodynamicFrc[N]/1
  Product2/1 -> MaxBrakeFrc[N]/1
  Add3/1 -> AverageRadius/1
  Add4/1 -> VehAndWheelInrtl[kg*m**2]/1
  Bus Selector/19 -> RoadSlopeLong[-]/1  "<VehicleRoadInfo_RoadSlopeLong[-]>"
  Abs/1 -> FinalDriveRatio[-]/1
  Bus Selector/1 -> Abs/1  "<VehicleDriverInfo_TorqueRatio[-]>"
  Bus Selector/3 -> Product/1, Product2/1, VehMass[kg]/1  "<VehicleDriverInfo_OverallMass[kg]>"
  Bus Selector/5 -> EngSpd[rad/s]/1  "<Drivetrain_DrivetrainPhysics_EngSpd[rad/s]>"
  Bus Selector/6 -> TractionCtrl/1(ClutchManual [0_1]), ClutchPos[0_1]/1  "<Drivetrain_DrivetrainPhysics_Clutch_Pos[0_1]>"
  Bus Selector/9 -> ExternalTrqs[Nm]/1  "<Auxiliaries_StarterTrq[Nm]>"
  Bus Selector/10 -> Add4/2  "<VehicleDriverInfo_SumWheelRotAxisInrt[kg*m**2]>"
  Bus Selector/11 -> Select x_value/1  "<Chassis_VehicleBody_AeroFrc(VehSys)[N]>"
  Select x_value/1 -> factor from vehicle data/1
  Bus Selector/12 -> SumMaxRollResistanceTrq[Nm]/1  "<VehicleDriverInfo_SumMaxRollingResistanceTrq[Nm]>"
  Bus Selector/13 -> Product2/2  "<VehicleDriverInfo_MaxDeceleration[m/s**2]>"
  Bus Selector/14 -> Add3/1  "<WheelSystem_FrontLeft_Tire_DynamicRadius[m]>"
  Bus Selector/15 -> Add3/2  "<WheelSystem_FrontRight_Tire_DynamicRadius[m]>"
  Bus Selector/16 -> Add3/3  "<WheelSystem_RearLeft_Tire_DynamicRadius[m]>"
  Bus Selector/17 -> Add3/4  "<WheelSystem_RearRight_Tire_DynamicRadius[m]>"
  Bus Selector/18 -> LongAeroDragCoeff[-]/1  "<VehicleDriverInfo_LongAeroDragCoeff[-]>"

== system PassengerCar/VehicleControl/LongitudinalControl/ControlSystems/Longitudinal Controller/Speed Control/Write to ControlOutputs ==
  AccPedalPos[0_1] : Inport
  IntendedEngTrq[Nm] : Inport  Port=2
  EngSpd[rad/s] : Inport  Port=3
  RefSpd[m/s] : Inport  Port=4
  RefAcc[m/s**2] : Inport  Port=5
  BrakePedalPos[0_1] : Inport  Port=6
  Bus Assignment : BusAssignment  AssignedSignals=AccPedalPos,BrakePedalPos,IntendedEngTrq,EngSpd,RefSpd,RefAcc
  Create SpeedControlOutput Bus : Constant  Value=0  OutDataTypeStr=Bus: TD_BO_LongitudinalSpeedControlOutputs
  ControlOutputs : Outport  VectorParamsAs1DForOutWhenUnconnected=off
  wires:
  RefSpd[m/s]/1 -> Bus Assignment/6  "RefSpd[m/s]"
  EngSpd[rad/s]/1 -> Bus Assignment/5  "EngSpd[rad/s]"
  IntendedEngTrq[Nm]/1 -> Bus Assignment/4  "IntendedEngTrq[Nm]"
  BrakePedalPos[0_1]/1 -> Bus Assignment/3  "BrakePedalPos[0_1]"
  AccPedalPos[0_1]/1 -> Bus Assignment/2  "AccPedalPos[0_1]"
  Bus Assignment/1 -> ControlOutputs/1
  Create SpeedControlOutput Bus/1 -> Bus Assignment/1
  RefAcc[m/s**2]/1 -> Bus Assignment/7  "RefAcc[m/s**2]"

== system PassengerCar/VehicleControl/LongitudinalControl/ControlSystemsPreprocessor/Generation of Speed Data/Smooth Derivative/Transfer Fcn with variable prameter ==
  note: Transfer function with variable parameters:
      | num = s
      | den = T^2*s^2 + 2*T*s + 1
      |
      | H(s) = Y(s) / U(s) = s / (T^2*s^2 + 2*T*s + 1)
      | -->
      | Y(s) = 1/T^2*1/s*U(s) - 2/T*1/s*Y(s) - 1/T^2*1/s^2*Y(s)
  u : Inport
  T : Inport  Port=2
  Add : Sum  Inputs=+--
  Discrete-Time Integrator : DiscreteIntegrator  InitialConditionSource=external  SampleTime=-1  ICPrevOutput=DiscIntNeverNeededParam  ICPrevScaledInput=DiscIntNeverNeededParam
  Discrete-Time Integrator1 : DiscreteIntegrator  InitialConditionSource=external  SampleTime=-1  ICPrevOutput=DiscIntNeverNeededParam  ICPrevScaledInput=DiscIntNeverNeededParam
  Discrete-Time Integrator2 : DiscreteIntegrator  SampleTime=-1  ICPrevOutput=DiscIntNeverNeededParam  ICPrevScaledInput=DiscIntNeverNeededParam
  Gain : Gain  Gain=2
  Gain2 : Gain  Gain=2
  Product1 : Product  Inputs=3
  Product2 : Product  Inputs=3
  Product3 : Product
  Product4 : Product
  Reciprocal : Product  Inputs=/
  y : Outport  VectorParamsAs1DForOutWhenUnconnected=off
  wires:
  Add/1 -> y/1, Discrete-Time Integrator1/1
  Product3/1 -> Gain/1
  T/1 -> Product4/2, Reciprocal/1
  Gain/1 -> Add/3
  Reciprocal/1 -> Product1/3, Product1/2, Product2/3, Product3/2, Product2/2
  Product2/1 -> Add/2
  Product1/1 -> Add/1
  Discrete-Time Integrator/1 -> Product1/1
  Discrete-Time Integrator2/1 -> Product2/1
  Discrete-Time Integrator1/1 -> Discrete-Time Integrator2/1, Product3/1
  Product4/1 -> Gain2/1
  u/1 -> Discrete-Time Integrator/1, Discrete-Time Integrator1/2, Product4/1
  Gain2/1 -> Discrete-Time Integrator/2

== system PassengerCar/VehicleControl/LateralControl/Disabled LateralControl/ControlSystems/Control Systems Parameters/CurvatureControl/DynaModuleInfo ==

== system PassengerCar/VehicleControl/LateralControl/Disabled LateralControl/ControlSystems/Control Systems Parameters/PathControl/DynaModuleInfo ==

== system PassengerCar/VehicleControl/LateralControl/Disabled LateralControl/ControlSystems/Lateral Controller/User-Defined Control/UserDefinedControl ==
  DynaModuleInfo : Subsystem  Tag=DynaModuleInfo
      mask init:
      | data = get_param(gcb, 'UserData');
      mask Display:
      | disp(['Type = ', data.type, '\nName = ', char(data.name)
      | ]);

== system PassengerCar/VehicleControl/LongitudinalControl/ControlSystems/Longitudinal Controller/Acceleration Control/ComputeBrakePedalPos/Calculate Brake Pedal ==
  Factor_TyreTorque_2_BrakePedalPosition : Inport
  Int Torque on Wheel : Inport  Port=2
  Constant1 : Constant  Value=0
  Divide : Product  Inputs=*/
  Gain : Gain  Gain=-1
  Limiter [0-1] : Subsystem
  Relational Operator : RelationalOperator  Operator=<  OutDataTypeStr=boolean  RndMeth=Nearest
  Switch : Switch  Threshold=0.5
  Brake Pedal Position : Outport  VectorParamsAs1DForOutWhenUnconnected=off
  wires:
  Limiter [0-1]/1(Out) -> Brake Pedal Position/1
  Int Torque on Wheel/1 -> Relational Operator/1, Gain/1
  Divide/1 -> Limiter [0-1]/1(In)
  Switch/1 -> Divide/1
  Gain/1 -> Switch/1
  Relational Operator/1 -> Switch/2
  Constant1/1 -> Switch/3, Relational Operator/2
  Factor_TyreTorque_2_BrakePedalPosition/1 -> Divide/2

== system PassengerCar/VehicleControl/LongitudinalControl/ControlSystems/Longitudinal Controller/Acceleration Control/ComputeBrakePedalPos/Factor_TyreTorque_2_BrakePedalPosition ==
  VehicleInfo : Inport
  Bus Selector3 : BusSelector  OutputSignals=VehicleDriverInfo_MaxMainBrakePress[Pa],WheelSystem_FrontLeft_Wheel_BrakeTrqPressRatio[m**3],WheelSystem_FrontRight_Wheel_BrakeTrqPressRatio[m**3],WheelSystem_RearLeft_Wheel_BrakeTrqPressRatio[m**3],WheelSystem_RearRight_Wheel_BrakeTrqPressRatio[m**3]
  Divide : Product  Inputs=**
  Sum of Elements : Sum  Inputs=++++
  Factor_TyreTorque_2_BrakePedalPosition : Outport  VectorParamsAs1DForOutWhenUnconnected=off
  wires:
  VehicleInfo/1 -> Bus Selector3/1
  Bus Selector3/1 -> Divide/1  "<VehicleDriverInfo_MaxMainBrakePress[Pa]>"
  Divide/1 -> Factor_TyreTorque_2_BrakePedalPosition/1
  Bus Selector3/2 -> Sum of Elements/1  "<WheelSystem_FrontLeft_Wheel_BrakeTrqPressRatio[m**3]>"
  Bus Selector3/3 -> Sum of Elements/2  "<WheelSystem_FrontRight_Wheel_BrakeTrqPressRatio[m**3]>"
  Bus Selector3/4 -> Sum of Elements/3  "<WheelSystem_RearLeft_Wheel_BrakeTrqPressRatio[m**3]>"
  Bus Selector3/5 -> Sum of Elements/4  "<WheelSystem_RearRight_Wheel_BrakeTrqPressRatio[m**3]>"
  Sum of Elements/1 -> Divide/2
